simulink model "UART_test"  (R2024b)
settings: Solver=FixedStepAuto  StartTime=0.0  StopTime=300  FixedStep=0.1  RelTol=1e-3  EnableMultiTasking=on
settings Model: ExtModeTrigDuration=2  Creator=USER  LastModifiedBy=USER
settings SolverCC: AutoInsertRateTranBlk=on
settings OptimizationCC: EnhancedBackFolding=on  PassReuseOutputArgsAs=Individual arguments  ZeroExternalMemoryAtStartup=off  ZeroInternalMemoryAtStartup=off  MaxStackSize=64  OptimizeBlockOrder=speed  DifferentSizesBufferReuse=on  OptimizationCustomize=off  EfficientTunableParamExpr=on
settings DebuggingCC: ParameterTunabilityLossMsg=error
settings HardwareCC: ProdBitPerInt=16  ProdBitPerPointer=16  ProdBitPerSizeT=16  ProdBitPerPtrDiffT=16  ProdLargestAtomicFloat=None  ProdWordSize=8  ProdHWDeviceType=Atmel->AVR
settings SFSimCC: MATLABDynamicMemAlloc=off
settings RTWCC: Description=Embedded Coder  SystemTargetFile=ert.tlc  HardwareBoard=Arduino Mega 2560  TemplateMakefile=ert_default_tmf  CustomHeaderCode="#include \"uart_handler.h\""  CustomInitializer=uart_init();  Toolchain=Arduino AVR  BuildConfiguration=Faster Runs
settings CodeAppCC: ForceParamTrailComments=on  IgnoreCustomStorageClasses=off  OperatorAnnotations=on  SimulinkDataObjDesc=on  SFDataObjDesc=on  InsertBlockDesc=on
settings ERTTargetCC: SupportContinuousTime=on  SupportVariableSizeSignals=on  ExtModeTransport=3  ExtModeStaticAlloc=on  ExtModeAutomaticAllocSize=off  ExtModeStaticAllocSize=2048  ExtModeMexFile=ext_xcp  ExtModeIntrfLevel=Level2 - Open  InlinedParameterPlacement=Hierarchical

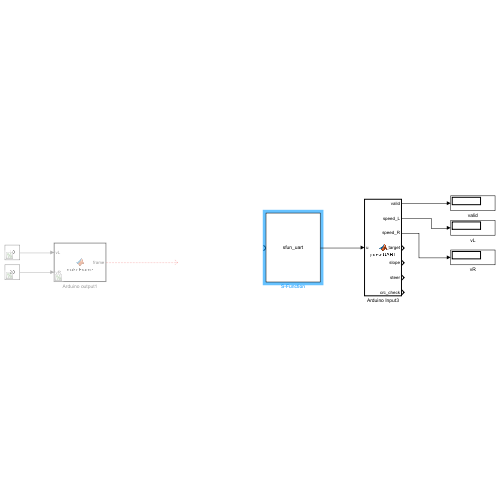
[thumbnail: Simulink's stored preview of the top-level diagram]
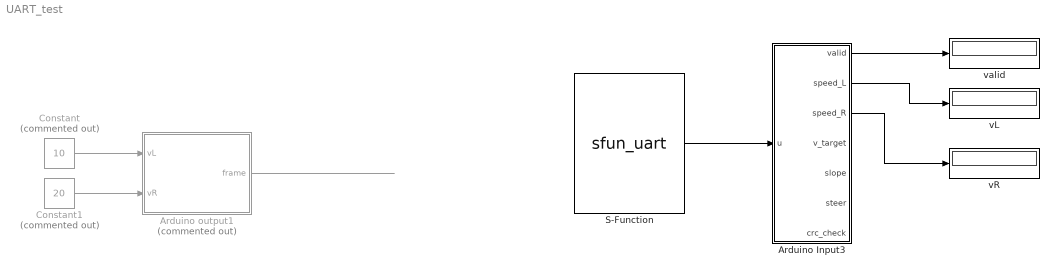
== system UART_test ==
  Arduino Input3 : MATLAB Function  TreatAsAtomicUnit=on
  Arduino output1 : MATLAB Function  Commented=on  TreatAsAtomicUnit=on
  Constant : Constant  Commented=on  Value=10
  Constant1 : Constant  Commented=on  Value=20
  S-Function : S-Function  FunctionName=sfun_uart  SFunctionDeploymentMode=off  EnableBusSupport=off
  vL : Display
  vR : Display
  valid : Display
  wires:
  Arduino output1/1(frame) -> ?
  S-Function/1 -> Arduino Input3/1(u)
  Arduino Input3/2(speed_L) -> vL/1
  Arduino Input3/1(valid) -> valid/1
  Constant/1 -> Arduino output1/1(vL)
  Constant1/1 -> Arduino output1/2(vR)
  Arduino Input3/3(speed_R) -> vR/1

== matlab function UART_test/Arduino Input3 ==
  data: valid output; speed_L output; speed_R output; v_target output; u input; slope output; steer output; crc_check output
function [valid, speed_L, speed_R, v_target, slope, steer, crc_check] = parseUART(u)

%#codegen

% 기본 출력 초기화
valid = uint8(0);
crc_check = uint8(0);
speed_L = double(0);
speed_R = double(0);
v_target = uint8(0);
slope = uint8(0);
steer = int8(0);

% 프레임 길이 및 헤더/테일 검사
`
if length(u) == 10 && u(1) == hex2dec('AA') && u(10) == hex2dec('55')

    % CRC 검사 (바이트 1~8까지 합 + CRC가 0 mod 256이어야 함)
    sum_payload = sum(double(u(1:8)));
    crc = double(u(9));

    if mod(sum_payload + crc, 256) == 0
        crc_check = uint8(1);
        valid = uint8(1);

        % 속도 L (정수 + 소수 / 100)
        speed_L = double(u(2)) + double(u(3)) / 100;

        % 속도 R (정수 + 소수 / 100)
        speed_R = double(u(4)) + double(u(5)) / 100;

        % 목표 속도
        v_target = u(6);

        % 경사각
        slope = u(7);

        % 조향각 (signed 처리)
        steer = typecast(uint8(u(8)), 'int8');  % 안전한 signed 변환
    end
end

end

== matlab function UART_test/Arduino output1 ==
  data: frame output; vL input; vR input
function frame = makeFrame(vL, vR)
% 입력:
%   vL, vR : 좌/우 목표 속도 (실수, cm/s 단위)
% 출력:
%   frame : 7-byte UART 전송 프레임 (uint8 벡터)
    frame = zeros(5,1,'uint8');  % 7바이트 프레임

    % 2-3. 목표속도_L (정수 + 소수)
    frame(1) = uint8(floor(vL));                       % 정수부
    frame(2) = uint8(floor(mod(vL * 100, 100)));       % 소수부 (소수점 둘째 자리까지)

    % 4-5. 목표속도_R (정수 + 소수)
    frame(3) = uint8(floor(vR));                       % 정수부
    frame(4) = uint8(floor(mod(vR * 100, 100)));       % 소수부

    % 6. CRC: 256 - (sum of byte 1~5) % 256
    crc = mod(sum(double(frame(1:5))), 256);
    frame(5) = uint8(mod(256 - crc, 256));
    
end
